simulink model "Converter"  (R2020a)
settings: Solver=ode45  StartTime=0.0  StopTime=10  RelTol=1e-3
libraries: powerlib x25, simulink x1, powerlib_meascontrol x1
settings Model: Creator=z_bhinde  LastModifiedBy=z_bhinde
settings SolverCC: ZeroCrossAlgorithm=Adaptive
settings DataIOCC: Refine=4
settings DebuggingCC: IgnoredZcDiagnostic=none

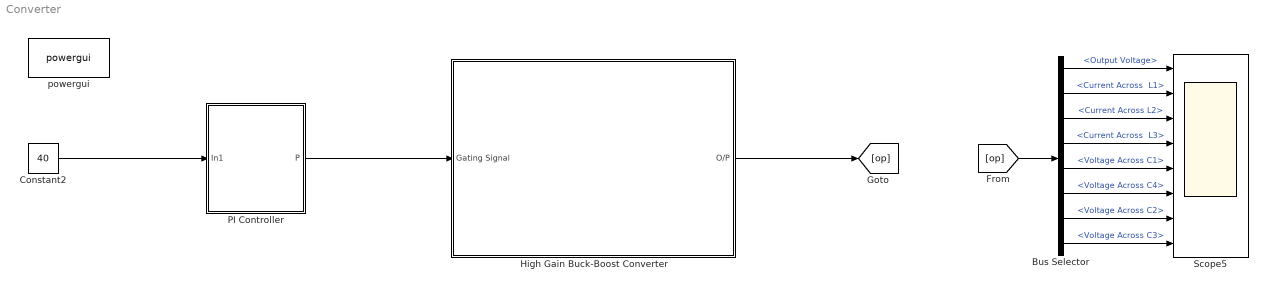
== system Converter ==
  Bus Selector : BusSelector  OutputSignals="Output Voltage,Current Across  L1,Current Across L2,Current Across  L3,Voltage Across C1,Voltage Across C4,Voltage Across C2,Voltage Across C3"
  Constant2 : Constant  Value=40
  High Gain Buck-Boost Converter : Subsystem  mask(High Gain Buck Boost Converter){C1=194.8e-6, C2=389.6e-6, C3=389.6e-6, C4=194.8e-6, L1=1.20585702e-3, L2=5.8079e-3, L3=5.8079e-3, Amplitude=11, Resistance=13.067}
      mask prompts: C1 "Capacitance  C1 (F):"; C2 "Capacitance C2 (F):"; C3 "Capacitance  C3 (F):"; C4 "Capacitance C4 (F):"; L1 "Inductance L1 (H):"; L2 "Inductance L2 (H):"; L3 "Inductance L3 (H):"; Amplitude "Input Voltage (V):"; Resistance "Output Resistance (Ohms):"
      mask help: This is a non-isolated transformerless high gain buck-boost dc-dc converter consisting of single switch. The designed converter gain is higher than other converters like buck-boost, boost, sepic, zeta and CUK converters.
      mask TypeOptions C1: C1/Capacitance
      mask TypeOptions C2: C2/Capacitance
      mask TypeOptions C3: C3/Capacitance
      mask TypeOptions C4: C4/Capacitance
      mask TypeOptions L1: L1/Inductance
      mask TypeOptions L2: L2/Inductance
      mask TypeOptions L3: L3/Inductance
      mask TypeOptions Amplitude: Vin/Amplitude
      mask TypeOptions Resistance: R1/Resistance
  PI Controller : Subsystem
  Scope5 : Scope  NumInputPorts=8
  powergui : powerlib/powergui  Priority=1  SimulationMode=Discrete  SampleTime=1e-6  frequency=60  Iterations=50  frequencyindice=0  Pbase=100e6  ErrMax=1e-4  UnitsV=kV  UnitsW=MW  buscounter=0  FunctionMessages=off  echomessages=off  EnableUseOfTLC=off  CurrentSourceSwitches=off  DisableSnubberDevices=off  DisableRonSwitches=off  DisableVfSwitches=off  DisplayEquations=off  AutomaticDiscreteSolvers=off  SolverType=Tustin/Backward Euler (TBE)  Interpol=off  ExternalGateDelay=off  methode=off  Ts=100  x0status=blocks  SPID=on  SwTol=0  HookPort=off  NonlinearTolerance=1e-4  nMaxIteration=100  ContinueOnMaxIteration=off  RestoreLinks=warning  ResistiveCurrentMeasurement=off  Frange=[0:2:500]  Ylog=off  Xlog=on  ShowGrid=off  save=off  variable=ZData  structure=0  ZoomFFT=off  StartTime=0.0  cycles=1  DisplayStyle=1  fundamental=60  FreqAxis=off  MaxFrequency=1000  frequencyindicesteady=1  RmsSteady=1  display=off
  wires:
  High Gain Buck-Boost Converter/1(O/P) -> [op]
  [op] -> Bus Selector/1
  Bus Selector/1 -> Scope5/1  "<Output Voltage>"
  Bus Selector/2 -> Scope5/2  "<Current Across  L1>"
  Bus Selector/3 -> Scope5/3  "<Current Across L2>"
  Bus Selector/4 -> Scope5/4  "<Current Across  L3>"
  Bus Selector/5 -> Scope5/5  "<Voltage Across C1>"
  Bus Selector/6 -> Scope5/6  "<Voltage Across C4>"
  Bus Selector/7 -> Scope5/7  "<Voltage Across C2>"
  Bus Selector/8 -> Scope5/8  "<Voltage Across C3>"
  Constant2/1 -> PI Controller/1(In1)
  PI Controller/1(P) -> High Gain Buck-Boost Converter/1(Gating Signal)

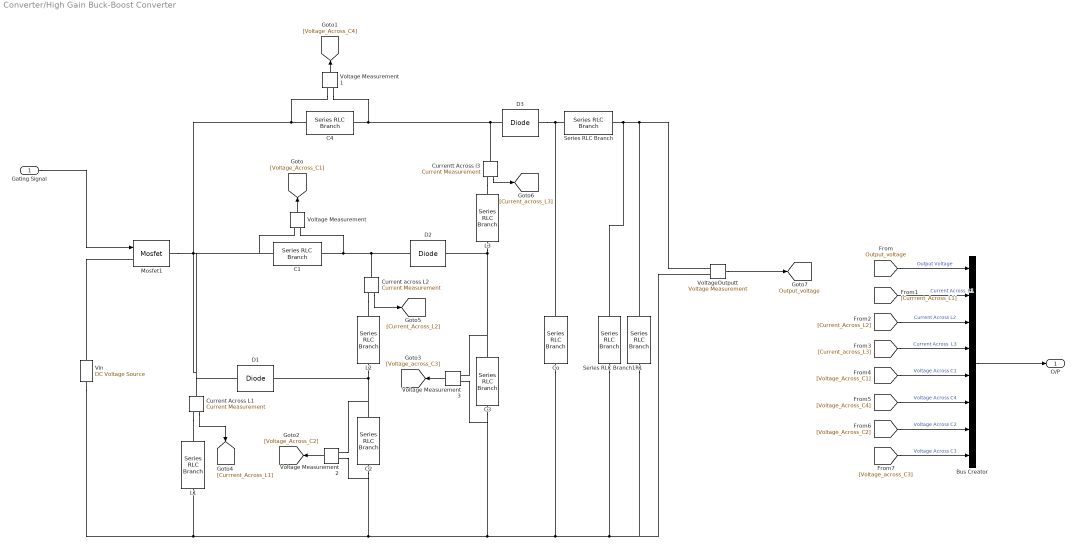
== system Converter/High Gain Buck-Boost Converter ==
  Gating Signal : Inport
  Bus Creator : BusCreator  Inputs=8
  C1 : powerlib/Elements/Series RLC Branch  LConnTagsString=__new0  RConnTagsString=__new0  BranchType=C  Resistance=1  Inductance=1e-3  SetiL0=off  InitialCurrent=0  Capacitance=C1  Setx0=off  InitialVoltage=0  Measurements=None
  C2 : powerlib/Elements/Series RLC Branch  LConnTagsString=__new0  RConnTagsString=__new0  BranchType=C  Resistance=1  Inductance=1e-3  SetiL0=off  InitialCurrent=0  Capacitance=C2  Setx0=off  InitialVoltage=0  Measurements=None
  C3 : powerlib/Elements/Series RLC Branch  LConnTagsString=__new0  RConnTagsString=__new0  BranchType=C  Resistance=1  Inductance=1e-3  SetiL0=off  InitialCurrent=0  Capacitance=C3  Setx0=off  InitialVoltage=0  Measurements=None
  C4 : powerlib/Elements/Series RLC Branch  LConnTagsString=__new0  RConnTagsString=__new0  BranchType=C  Resistance=1  Inductance=1e-3  SetiL0=off  InitialCurrent=0  Capacitance=C4  Setx0=off  InitialVoltage=0  Measurements=None
  Co : powerlib/Elements/Series RLC Branch  LConnTagsString=__new0  RConnTagsString=__new0  BranchType=C  Resistance=1  Inductance=1e-3  SetiL0=off  InitialCurrent=0  Capacitance=800e-6  Setx0=off  InitialVoltage=0  Measurements=None
  Current Across L1 : powerlib/Measurements/Current Measurement  PhasorSimulation=off  OutputType=Complex  PSBequivalent=0
  Current across L2 : powerlib/Measurements/Current Measurement  PhasorSimulation=off  OutputType=Complex  PSBequivalent=0
  Currentt Across l3 : powerlib/Measurements/Current Measurement  PhasorSimulation=off  OutputType=Complex  PSBequivalent=0
  D1 : powerlib/Power Electronics/Diode  Ron=1e-6  Lon=0  Vf=0.8  IC=0  UseSnubber=0  Rs=500  Cs=250e-9  Measurements=off
  D2 : powerlib/Power Electronics/Diode  Ron=1e-6  Lon=0  Vf=0.8  IC=0  UseSnubber=0  Rs=500  Cs=250e-9  Measurements=off
  D3 : powerlib/Power Electronics/Diode  Ron=1e-6  Lon=0  Vf=0.8  IC=0  UseSnubber=0  Rs=500  Cs=250e-9  Measurements=off
  L1 : powerlib/Elements/Series RLC Branch  LConnTagsString=__new0  RConnTagsString=__new0  BranchType=L  Resistance=1  Inductance=L1  SetiL0=off  InitialCurrent=0  Capacitance=1e-6  Setx0=off  InitialVoltage=0  Measurements=None
  L2 : powerlib/Elements/Series RLC Branch  LConnTagsString=__new0  RConnTagsString=__new0  BranchType=L  Resistance=1  Inductance=L2  SetiL0=off  InitialCurrent=0  Capacitance=1e-6  Setx0=off  InitialVoltage=0  Measurements=None
  L3 : powerlib/Elements/Series RLC Branch  LConnTagsString=__new0  RConnTagsString=__new0  BranchType=L  Resistance=1  Inductance=L3  SetiL0=off  InitialCurrent=0  Capacitance=1e-6  Setx0=off  InitialVoltage=0  Measurements=None
  Mosfet1 : powerlib/Power Electronics/Mosfet  Ron=0.1e-6  Lon=0  Rd=0.1e-6  Vfd=0  IC=0  Rs=1e5  Cs=inf  Measurements=off
  R1 : powerlib/Elements/Series RLC Branch  LConnTagsString=__new0  RConnTagsString=__new0  BranchType=R  Resistance=Resistance  Inductance=1e-3  SetiL0=off  InitialCurrent=0  Capacitance=1e-6  Setx0=off  InitialVoltage=0  Measurements=None
  Series RLC Branch : powerlib/Elements/Series RLC Branch  LConnTagsString=__new0  RConnTagsString=__new0  BranchType=L  Resistance=1  Inductance=100e-9  SetiL0=off  InitialCurrent=0  Capacitance=1e-6  Setx0=off  InitialVoltage=0  Measurements=None
  Series RLC Branch1 : powerlib/Elements/Series RLC Branch  LConnTagsString=__new0  RConnTagsString=__new0  BranchType=C  Resistance=1  Inductance=100e-9  SetiL0=off  InitialCurrent=0  Capacitance=33e-6  Setx0=off  InitialVoltage=0  Measurements=None
  Vin : powerlib/Electrical Sources/DC Voltage Source  Amplitude=Amplitude  Measurements=None
  Voltage Measurement{,1..3} (4 alike) : powerlib/Measurements/Voltage Measurement  PhasorSimulation=off  OutputType=Complex  PSBequivalent=0
  VoltageOutputt : powerlib/Measurements/Voltage Measurement  PhasorSimulation=off  OutputType=Complex  PSBequivalent=0
  O/P : Outport
  tag scope: Output_voltage=global
  wires:
  Gating Signal/1 -> Mosfet1/1
  Voltage Measurement/1 -> [Voltage_Across_C1]
  Voltage Measurement1/1 -> [Voltage_Across_C4]
  Voltage Measurement2/1 -> [Voltage_Across_C2]
  Voltage Measurement3/1 -> [Voltage_across_C3]
  Current Across L1/1 -> [Currrent_Across_L1]
  Current across L2/1 -> [Current_Across_L2]
  Currentt Across l3/1 -> [Current_across_L3]
  VoltageOutputt/1 -> [Output_voltage]
  [Output_voltage] -> Bus Creator/1  "Output Voltage"
  [Currrent_Across_L1] -> Bus Creator/2  "Current Across  L1"
  [Current_Across_L2] -> Bus Creator/3  "Current Across L2"
  [Current_across_L3] -> Bus Creator/4  "Current Across  L3"
  [Voltage_Across_C1] -> Bus Creator/5  "Voltage Across C1"
  [Voltage_Across_C4] -> Bus Creator/6  "Voltage Across C4"
  [Voltage_Across_C2] -> Bus Creator/7  "Voltage Across C2"
  [Voltage_across_C3] -> Bus Creator/8  "Voltage Across C3"
  Bus Creator/1 -> O/P/1
  connections:
  L2/RConn1 -- Voltage Measurement2/LConn2 -- C2/RConn1 -- D1/LConn1
  Vin/LConn1 -- Voltage Measurement2/LConn1 -- C2/LConn1 -- Voltage Measurement3/LConn1 -- C3/LConn1 -- R1/LConn1 -- VoltageOutputt/LConn1 -- Series RLC Branch1/LConn1 -- Co/LConn1 -- L1/RConn1
  D2/RConn1 -- Current across L2/LConn1 -- Voltage Measurement/LConn2 -- C1/RConn1
  D3/LConn1 -- Series RLC Branch/LConn1 -- Co/RConn1
  D3/RConn1 -- Currentt Across l3/LConn1 -- Voltage Measurement1/LConn2 -- C4/RConn1
  C4/LConn1 -- Mosfet1/RConn1 -- Voltage Measurement/LConn1 -- C1/LConn1 -- Current Across L1/LConn1 -- D1/RConn1 -- Voltage Measurement1/LConn1
  L3/RConn1 -- Voltage Measurement3/LConn2 -- C3/RConn1 -- D2/LConn1
  Currentt Across l3/RConn1 -- L3/LConn1
  Current Across L1/RConn1 -- L1/LConn1
  Mosfet1/LConn1 -- Vin/RConn1
  Current across L2/RConn1 -- L2/LConn1
  Series RLC Branch/RConn1 -- Series RLC Branch1/RConn1 -- R1/RConn1 -- VoltageOutputt/LConn2

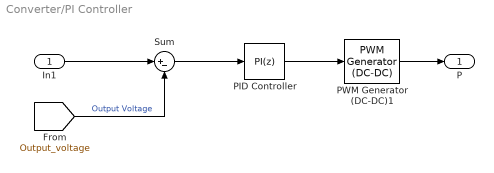
== system Converter/PI Controller ==
  In1 : Inport
  PID Controller : simulink/Continuous/PID Controller  Controller=PI  Form=Parallel  TimeDomain=Discrete-time  UseExternalTs=off  SampleTime=-1  IntegratorMethod=Forward Euler  FilterMethod=Forward Euler  ControllerParametersSource=internal  P=0.000330956716472386  I=0.043886369479558  D=0  UseFilter=on  N=100  TunerSelectOption=Transfer Function Based (PID Tuner App)  InitialConditionSource=internal  InitialConditionForIntegrator=0  InitialConditionForFilter=0  DifferentiatorICPrevScaledInput=0  ExternalReset=none  TrackingMode=off  Kt=1  LimitOutput=off  UpperSaturationLimit=inf  LowerSaturationLimit=-inf  LinearizeAsGain=on  AntiWindupMode=none  Kb=1  POutMin=[]  POutMax=[]  IOutMin=[]  IOutMax=[]  DOutMin=[]  DOutMax=[]  NOutMin=[]  NOutMax=[]  SumOutMin=[]  SumOutMax=[]  SaturationOutMin=[]  SaturationOutMax=[]  PParamMin=[]  PParamMax=[]  IParamMin=[]  IParamMax=[]  DParamMin=[]  DParamMax=[]  NParamMin=[]  NParamMax=[]  KbParamMin=[]  KbParamMax=[]  KtParamMin=[]  KtParamMax=[]  KbOutMin=[]  KbOutMax=[]  KtOutMin=[]  KtOutMax=[]  IntegratorOutMin=[]  IntegratorOutMax=[]  FilterOutMin=[]  FilterOutMax=[]  SumI1OutMin=[]  SumI1OutMax=[]  SumI2OutMin=[]  SumI2OutMax=[]  SumI3OutMin=[]  SumI3OutMax=[]  SumI4OutMin=[]  SumI4OutMax=[]  SumDOutMin=[]  SumDOutMax=[]  DifferentiatorOutMin=[]  DifferentiatorOutMax=[]  FilterDiffOutCoefMin=[]  FilterDiffOutCoefMax=[]  ReciprocalOutMin=[]  ReciprocalOutMax=[]  SumDenOutMin=[]  SumDenOutMax=[]  SumNumOutMin=[]  SumNumOutMax=[]  DivideOutMin=[]  DivideOutMax=[]  UdiffTsProdOutMin=[]  UdiffTsProdOutMax=[]  NTsProdOutMin=[]  NTsProdOutMax=[]  UintegralTsProdOutMin=[]  UintegralTsProdOutMax=[]  UngainTsProdOutMin=[]  UngainTsProdOutMax=[]  IntegratorContinuousStateAttributes=''  IntegratorStateMustResolveToSignalObject=off  IntegratorRTWStateStorageClass=Auto  FilterContinuousStateAttributes=''  FilterStateMustResolveToSignalObject=off  FilterRTWStateStorageClass=Auto  ParallelPVariant=InternalParameters  IdealPVariant=Disabled  IVariant=InternalParameters  DVariant=Disabled  IntegratorVariant=Discrete  SatVariant=Disabled  AWVariant=Passthrough  PCopyVariant=Disabled  TRVariant=Disabled  FdbkBlocksVariant=Forward  IdealPFdbkVariant=Disabled  SatFdbkVariant=Disabled  DerivativeFilterVariant=Disabled  NVariant=Disabled  NCopyVariant=Disabled_SignalSpec  FilterICVariant=Disabled  IntegratorICVariant=InternalICs  ExternalResetVariant=Disabled  TRSumVariant=Passthrough  SumFdbkVariant=Disabled  SumVariant=Sum_PI  TsampFilterVariant=InternalTs  TsampNgainVariant=Passthrough  TsampIntegralVariant=Passthrough
  PWM Generator (DC-DC)1 : powerlib_meascontrol/Pulse & Signal Generators/PWM Generator (DC-DC)  Fsw=33000  Ts=0
  Sum : Sum  Inputs=|+-
  P : Outport
  wires:
  PID Controller/1 -> PWM Generator (DC-DC)1/1
  In1/1 -> Sum/1
  Sum/1 -> PID Controller/1
  PWM Generator (DC-DC)1/1 -> P/1
  [Output_voltage] -> Sum/2  "Output Voltage"
